simulink model "testsim"  (R2019b)
settings: Solver=ode14x  StartTime=0.0  StopTime=500  FixedStep=0.01  RelTol=1e-3
settings Model: Creator=Administrator  LastModifiedBy=Administrator

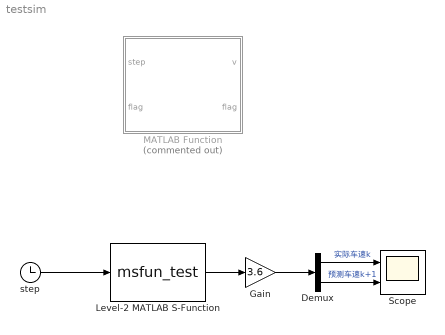
== system testsim ==
  Demux : Demux  Outputs=2
  Gain : Gain  Gain=3.6
  Level-2 MATLAB S-Function : M-S-Function  FunctionName=msfun_test
  MATLAB Function : MATLAB Function  Commented=on  TreatAsAtomicUnit=on
  Scope : Scope  NumInputPorts=2
  step : Clock
  wires:
  Demux/2 -> Scope/2  "预测车速k+1"
  step/1 -> Level-2 MATLAB S-Function/1
  Level-2 MATLAB S-Function/1 -> Gain/1
  Demux/1 -> Scope/1  "实际车速k"
  Gain/1 -> Demux/1

== matlab function testsim/MATLAB Function ==
  data: step input; v output; flag input; flag output
function [v,flag] = fcn(step,flag)
    scenarioPath='D:/BaiduNetdiskDownload/sumo-win64extra-1.8.0/sumo-1.8.0/file/MATLAB_QKJ/1.sumocfg';
    traci.start(['sumo-gui -c ' '"' scenarioPath '"' ' --start']);
if flag==1
    step=step;
    v=traci.vehicle.getSpeed('vehicle_0');
    traci.simulation.step()
else
    step=step;
    v=traci.vehicle.getSpeed('vehicle_0');
    traci.simulation.step()
end
flag=0;
